simulink model "ftm_dual_edge_s32k14x"  (Simulink 9.0)
settings: Solver=FixedStepDiscrete  StartTime=0.0  StopTime=10.0  FixedStep=1  RelTol=1e-3  EnableMultiTasking=on
InitFcn:
  | mbd_s32k_consistency_checks(bdroot(gcs));
undefined symbols (not defined in the file): LQFP, One, Shot
libraries: mbd_s32k1xx_ec_toolbox x9, simulink x1
Description:
  | This model shows FlexTimer Dual Edge Capture Mode.
  | Connect FTM0 Channel 0 output  PTC0 (J4.11) to FTM2 Channel 4 input PTD13 (J2.1).
  | Connect FTM0 Channel 1 output PTC1 (J5.13) to FTM2 Channel 6 input PTE15 (J5.4).
  | 
  | FTM2 channel 4 interrupt measures Period width of PTC0 10 kHz output  and toggles
  | PTA16 (J5.3) pin at every its Rising edge.
  | FTM2 channel 6 interrupt measures Positive Pulse width of PTC1 10 kHz 30% duty-cycle
  | output and toggles PTA15 (J5.1) pin at every its Falling edge.
  | 
  | Validation:
  | - Measured Pulse and Period values by FreeMaster using ftm_dual_edge_s32k14.pmp
settings Model: Creator=NXP MBDT Team  LastModifiedBy=nxf35172
settings DataIOCC: ExternalInput=off  InitialState=off  LimitDataPoints=on  SaveOutput=off  SignalLogging=off  SaveTime=off
settings OptimizationCC: DefaultParameterBehavior=Inlined  LifeSpan=1
settings DebuggingCC: SolverPrmCheckMsg=warning  InheritedTsInSrcMsg=none  SingleTaskRateTransMsg=error  UnconnectedInputMsg=error  UnconnectedOutputMsg=error  UnconnectedLineMsg=error  AllowSymbolicDim=off  UnknownTsInhSupMsg=error  StateNameClashWarn=warning
settings HardwareCC: ProdLargestAtomicInteger=Long  ProdLargestAtomicFloat=Double  ProdEndianess=LittleEndian  ProdHWDeviceType=ARM Compatible->ARM Cortex
settings SFSimCC: MATLABDynamicMemAlloc=off
settings RTWCC: SystemTargetFile=mbd_s32k.tlc  MakeCommand=mbd_s32k_make_rtw COPY_MDLREF_INCLUDES=0  TemplateMakefile=mbd_s32k.tmf  Description=Model Based Design Toolbox S32K14x Code Generation Target  GenerateReport=on  IncludeHyperlinkInReport=on  LaunchReport=on
settings CodeAppCC: IgnoreCustomStorageClasses=off
settings STFCustomTargetCC: CombineOutputUpdateFcns=on  ERTCustomFileBanners=on  SupportContinuousTime=off  SupportNonInlinedSFcns=off  RemoveResetFunc=on  MATLABClassNameForMDSCustomization=Simulink.SoftwareTarget.ERTCustomization  GRTInterface=off  SystemTargetFile=mbd_s32k14.tlc
settings ERTTargetCC: MultiwordLength=2048  ParMdlRefBuildCompliant=off  CompOptLevelCompliant=off  ConcurrentExecutionCompliant=off  ModelStepFunctionPrototypeControlCompliant=off  CPPClassGenCompliant=off  UseToolchainInfoCompliant=off  InlinedParameterPlacement=NonHierarchical  ERTCustomFileTemplate=example_file_process.tlc  ConvertIfToSwitch=off  SuppressUnreachableDefaultCases=off

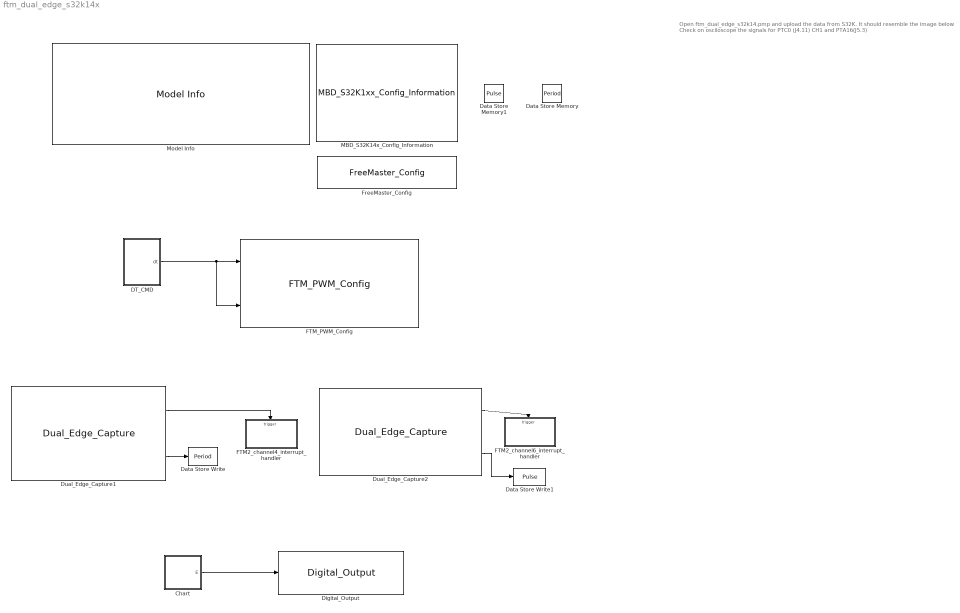
== system ftm_dual_edge_s32k14x ==
  note: Open ftm_dual_edge_s32k14.pmp and upload the data from S32K. It should resemble the image below
      |
      | Check on osciloscope the signals for PTC0 (J4.11) CH1 and PTA16(J5.3)
  Chart : Stateflow chart  TreatAsAtomicUnit=on
  DT_CMD : Stateflow chart  Priority=0  TreatAsAtomicUnit=on
  Data Store Memory : DataStoreMemory  DataStoreName=Period  ReadBeforeWriteMsg=warning  WriteAfterWriteMsg=warning  WriteAfterReadMsg=warning  ShowAdditionalParam=off  OutDataTypeStr=uint16
  Data Store Memory1 : DataStoreMemory  DataStoreName=Pulse  ReadBeforeWriteMsg=warning  WriteAfterWriteMsg=warning  WriteAfterReadMsg=warning  ShowAdditionalParam=off  OutDataTypeStr=uint16
  Data Store Write : DataStoreWrite  DataStoreName=Period
  Data Store Write1 : DataStoreWrite  DataStoreName=Pulse
  Digital_Output : mbd_s32k1xx_ec_toolbox/GPIO Blocks/Digital_Output  gpio_pin=PTD0: [PTD0 | Port D I/O]  init_val=Low  drive_strength=Low
  Dual_Edge_Capture1 : mbd_s32k1xx_ec_toolbox/Motor Control Blocks/FTM Blocks/Dual_Edge_Capture  Priority=2  ftmModule=2  channel=4-5  c_mode=One-Shot  mesur=period (rising - rising)  prescaler=1  filter_en=off  filter_value=0  isrlevel=12  pinFtmCh=PTD13: [FTM2_CH4 | FTM Channel]
  Dual_Edge_Capture2 : mbd_s32k1xx_ec_toolbox/Motor Control Blocks/FTM Blocks/Dual_Edge_Capture  Priority=3  ftmModule=2  channel=6-7  c_mode=Continuous  mesur=positive pulse (rising - falling)  prescaler=1  filter_en=off  filter_value=0  isrlevel=12  pinFtmCh=PTE15: [FTM2_CH6 | FTM Channel]
  FTM2_channel4_interrupt_handler : Subsystem  TreatAsAtomicUnit=on
      settings: RTWSystemCode=Nonreusable function
  FTM2_channel6_interrupt_handler : Subsystem  TreatAsAtomicUnit=on
      settings: RTWSystemCode=Nonreusable function
  FTM_PWM_Config : mbd_s32k1xx_ec_toolbox/Motor Control Blocks/FTM Blocks/FTM_PWM_Config  Priority=1  ftmModule=0  ftmMode=Edge-Aligned PWM  ftmSourceClock=80 MHz  swcontrol_enable=off  chan0En=on  chan0Type=Independent  chan2En=off  chan2Type=Independent  chan4En=off  chan4Type=Independent  chan6En=off  chan6Type=Independent  ftmPwmUnits=Hz  outFrequency=10000  ftmPeriod=8000  ftmPrescaler=Divide by 1  deadtimeUnits=Nanoseconds  deadtimeNs=0  deadtimeTicks=0  deadtimePrescaler=Divide by 1  dutyCycleCh0=0.5  dutyCycleCh1=0.5  dutyCycleCh2=0.25  dutyCycleCh3=0.25  dutyCycleCh4=0.25  dutyCycleCh5=0.25  dutyCycleCh6=0.25  dutyCycleCh7=0.25  dutyCycleSim=off  startAfterInit=on  showAdvOpt=on  pinFtmCh0=PTC0: [FTM0_CH0 | FTM Channel]  pinFtmCh1=PTC1: [FTM0_CH1 | FTM Channel]  pinPolCh0=Active Low  pinPolCh1=Active High  outputComplem0=Main duplicated  outputLevel0=Low  outputLevel1=Low  pinFtmCh2=PTB14: [FTM0_CH2 | FTM Channel]  pinFtmCh3=None  pinPolCh2=Active Low  pinPolCh3=Active Low  outputComplem2=Main duplicated  outputLevel2=Low  outputLevel3=Low  pinFtmCh4=PTB4: [FTM0_CH4 | FTM Channel]  pinFtmCh5=None  pinPolCh4=Active Low  pinPolCh5=Active Low  outputComplem4=Main duplicated  outputLevel4=Low  outputLevel5=Low  pinFtmCh6=PTA17: [FTM0_CH6 | FTM Channel]  pinFtmCh7=None  pinPolCh6=Active Low  pinPolCh7=Active Low  outputComplem6=Main duplicated  outputLevel6=Low  outputLevel7=Low  initTrigger=off  chTrigger0=off  chTrigger1=off  chTrigger2=off  chTrigger3=off  chTrigger4=off  chTrigger5=off  chTrigger6=off  chTrigger7=off  mcuTargetUpdate=on  pwmSyncTrg=Software trigger  pwmSyncHwRouting=TRGMUX_FTM7  pwmSyncTrg0=off  pwmSyncTrg1=off  pwmSyncTrg2=off  pwmSyncAutoClear=on  pwmSyncMinLoad=on  pwmSyncMaxLoad=on  pwmSyncInvert=System Clock  pwmSyncOutControl=System Clock  pwmSyncOutMask=System Clock  pwmSyncCounterInitial=System Clock  pwmSyncPoints=Update now  reloadEnable=off  reloadPriority=15  reloadHalfCycle=off  reloadHCR=0  reloadFrequency=0  chnMatch0=off  chnMatch1=off  chnMatch2=off  chnMatch3=off  chnMatch4=off  chnMatch5=off  chnMatch6=off  chnMatch7=off  pwmFaultProtection=off  pwmFaultInterrupt=off  pwmFaultClearing=Fault control disabled  pwmFaultPinState=Safe Value  pwmFaultFilterValue=0  pwmFaultPriority=15  fault_disen_0=off  fault_filter_0=off  fault_polarity_0=Active High  fault_disen_1=off  fault_filter_1=off  fault_polarity_1=Active high  fault_disen_2=off  fault_filter_2=off  fault_polarity_2=Active high  fault_disen_3=off  fault_filter_3=off  fault_polarity_3=Active high  fault_pin_0=None  fault_pin_1=None  fault_pin_2=None  fault_pin_3=None
  FreeMaster_Config : mbd_s32k1xx_ec_toolbox/Utility Blocks/FreeMaster_Config  interface=LPUART1  baudrate=115200  rxd=PTC6: [LPUART1_RX | Receive]  txd=PTC7: [LPUART1_TX | Transmit]  mode=Short Interrupt  isr_prio=15  show_adv_opts=off  use_scope=on  max_scope_vars=8  use_recorder=on  max_rec_vars=8  rec_buff_size=1024  rec_timebase=0 milliseconds  comm_buffer_size_auto=on  comm_buffer_size=255  comm_rqueue_size_default=on  comm_rqueue_size=32
  MBD_S32K14x_Config_Information : mbd_s32k1xx_ec_toolbox/MBD_S32K1xx_Config_Information  Priority=0  mbdt_ver=0  disp_str=|  config_params=[]  mcu_target_name=S32K144  mcu_target_package=64-LQFP  mcu_target_sram_size=48KB  mcu_system_clock_freq=80  mcu_xtal_freq=External 8  mcu_steptick_timer=LPIT Channel 0  mcu_steptick_prio=15  ds_import_enable=on  target_compiler=GCC  target_memory=FLASH  gcc_target_compile_opts=-mcpu=cortex-m4 -mthumb -mfloat-abi=hard -mfpu=fpv4-sp-d16 -O1 -g -gstrict-dwarf  gcc_target_assemble_opts=-mcpu=cortex-m4 -mthumb -mfloat-abi=hard -mfpu=fpv4-sp-d16 -g  gcc_target_link_opts=-mcpu=cortex-m4 -mthumb -mfloat-abi=hard -mfpu=fpv4-sp-d16  gcc_target_default_lcf=on  gcc_target_user_lcf=S32K144_48_flash.ld  ghs_target_compile_opts=-cpu=cortexm4f -thumb -DARM_MATH_CM4 -fpu=vfpv4_d16 -fsingle -Ogeneral -Wundef -Wimplicit-int -Wshadow -Wtrigraphs --no_commons --gnu_asm -gnu99 -gdwarf-2 -G  ghs_target_assemble_opts=-cpu=cortexm4f -fpu=vfpv4_d16  ghs_target_link_opts=-cpu=cortexm4f -thumb -fpu=vfpv4_d16  ghs_target_default_lcf=off  ghs_target_user_lcf=S32K144_48_flash.ld  iar_target_compile_opts=--cpu=Cortex-M4F --thumb --fpu=VFPv4_sp -Ol -e --debug --dlib_config normal  iar_target_assemble_opts=--cpu Cortex-M4F --thumb --fpu VFPv4_sp  iar_target_link_opts=--no_exceptions --vfe --inline  iar_target_default_lcf=off  iar_target_user_lcf=S32K144_48_flash.icf  pil_download_enable=off  rbl_download_enable=on  rbl_start_delay=5000000  rbl_download_interface=OpenSDA  rbl_restart_request=off  rbl_com_port=Custom  rbl_com_port_custom=COM1  pil_download_rate=57600  pil_opensda_drive=Custom  pil_opensda_drive_custom=D  pil_uart_instance=0  pil_uart_rx=PTA2: [LPUART0_RX | Receive]  pil_uart_tx=PTA3: [LPUART0_TX | Transmit]  FTM_PWM_PcrCheckEnDis=on  FTM_Input_Edge_Inputs_PcrCheckEnDis=on  FTM_Dual_Edge_Inputs_PcrCheckEnDis=on  FTM_Quadrature_Inputs_PcrCheckEnDis=on  FTM_Hall_Sensor_Inputs_PcrCheckEnDis=on  LPTMR_PcrCheckEnDis=on  PIT_PcrCheckEnDis=on  RTC_PcrCheckEnDis=on  FlexCAN_PcrCheckEnDis=on  LIN_PcrCheckEnDis=on  FlexIO_PcrCheckEnDis=on  LPI2C_PcrCheckEnDis=on  LPSPI_PcrCheckEnDis=on  LPUART_PcrCheckEnDis=on  CMP_PcrCheckEnDis=on  GPIO_OutputPcrCheckEnDis=on  GPIO_InputPcrCheckEnDis=on  SBC_PcrCheckEnDis=on  AMMCLIB_PcrCheckEnDis=on  FM_PcrCheckEnDis=on  Profile_PcrCheckEnDis=on  ConfigParams_PcrCheckEnDis=on  ModelRef_PcrCheckEnDis=on  PDB0_PcrCheckEnDis=on  CSEc_PcrCheckEnDis=on  eDMA_PcrCheckEnDis=on  ADC_PcrCheckEnDis=on  WDOG_PcrCheckEnDis=on
      | Target : S32K142-16KB_SRAM
      | Package : 100-pin
      | System clock : 80 MHz
      | XTAL clock : External 8 MHz
      | Compiler : GCC
      | Target Type : FLASH
      | Download Code after build : (OpenSDA: E)
      | Step Tick Interrupt Priority : 15
  Model Info : simulink/Model-Wide Utilities/Model Info  Frame=off  DisplayStringWithTags=|  HorizontalTextAlignment=Left  LeftAlignmentValue=0.02
      | Model Name: %<ModelName>
      | 
      | Description: %<Description>
  wires:
  DT_CMD/1(dt) -> FTM_PWM_Config/2, FTM_PWM_Config/1
  Dual_Edge_Capture1/1 -> FTM2_channel4_interrupt_handler/Trigger
  Dual_Edge_Capture2/2 -> Data Store Write1/1
  Dual_Edge_Capture2/1 -> FTM2_channel6_interrupt_handler/Trigger
  Dual_Edge_Capture1/2 -> Data Store Write/1
  Chart/1(" E") -> Digital_Output/1

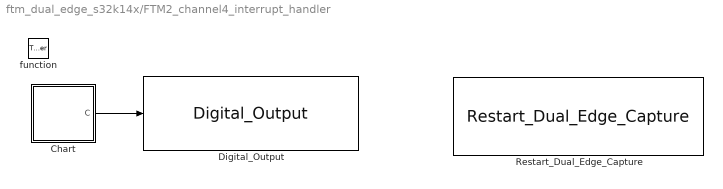
== system ftm_dual_edge_s32k14x/FTM2_channel4_interrupt_handler ==
  function : TriggerPort  TriggerType=function-call  VariantControl=Variant
  Chart : Stateflow chart  TreatAsAtomicUnit=on
  Digital_Output : mbd_s32k1xx_ec_toolbox/GPIO Blocks/Digital_Output  gpio_pin=PTA16: [PTA16 | Port A I/O]  init_val=Low  drive_strength=Low
  Restart_Dual_Edge_Capture : mbd_s32k1xx_ec_toolbox/Motor Control Blocks/FTM Blocks/Restart_Dual_Edge_Capture  Priority=1  ftmModule=2  channel=4-5
  wires:
  Chart/1(" C") -> Digital_Output/1

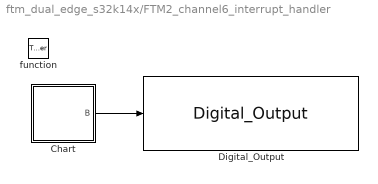
== system ftm_dual_edge_s32k14x/FTM2_channel6_interrupt_handler ==
  function : TriggerPort  TriggerType=function-call  VariantControl=Variant
  Chart : Stateflow chart  TreatAsAtomicUnit=on
  Digital_Output : mbd_s32k1xx_ec_toolbox/GPIO Blocks/Digital_Output  gpio_pin=PTA15: [PTA15 | Port A I/O]  init_val=Low  drive_strength=Low
  wires:
  Chart/1(" B") -> Digital_Output/1

== stateflow chart FTM2_channel4_interrupt_handler/Chart ==
  state C
  state C1
  (default) -> C
  C -> C1
  C1 -> C
  data: C output boolean [0..1]

== stateflow chart DT_CMD ==
  settings: executeAtInitialization=1
  state A
    du:
    dt =0.3;
    cntr=cntr+1;
  state A1
    du:
    dt =0.6;
    cntr=cntr-1;
  (default) -> A : {cntr=0;}
  A1 -> A : [cntr < 1]
  A -> A1 : [cntr > 5]
  data: cntr local uint32 =0; dt output single

== stateflow chart FTM2_channel6_interrupt_handler/Chart ==
  state B
  state B1
  (default) -> B
  B -> B1
  B1 -> B
  data: B output boolean [0..1]

== stateflow chart Chart ==
  state E
  state E1
  (default) -> E
  E -> E1
  E1 -> E
  data: E output boolean [0..1]
